simulink model "RNEDynamics"  (R2022b)
settings: Solver=ode23  StartTime=0.0  StopTime=tSim  RelTol=1e-3
values from neighbouring files (symbols this model uses):
  KdInner = 20 * eye(6)    [main.m]    (also in mainJoint.m = 40 * eye(6))
  KpInner = 4 * eye(6)    [main.m]    (also in mainJoint.m)
  qdotIC = [0, 0, 0, 0, 0, 0]'    [mainJoint.m]
  qIC = theta0'    [mainJoint.m]
  Robot = SerialLink(L)    [main.m]    (also in mainJoint.m)
undefined symbols (not defined in the file or in its folder): calcTorques, manipulatorPlant
libraries: sldrtlib x1
settings Model: Creator=Hunter  LastModifiedBy=Hunter
settings HardwareCC: ProdBitPerLong=64  ProdHWDeviceType=Intel->x86-64 (Linux 64)
settings RTWCC: Description=Simulink Desktop Real-Time  SystemTargetFile=sldrt.tlc  TemplateMakefile=sldrt.tmf  RTWCompilerOptimization=on
settings CodeAppCC: MaxIdLength=95
settings SimulinkDesktopRealTimeCC: TargetLibSuffix=_sldrt.a  TargetPreCompLibLocation=C:\Program Files\MATLAB\R2022b\toolbox\sldrt\lib\win64

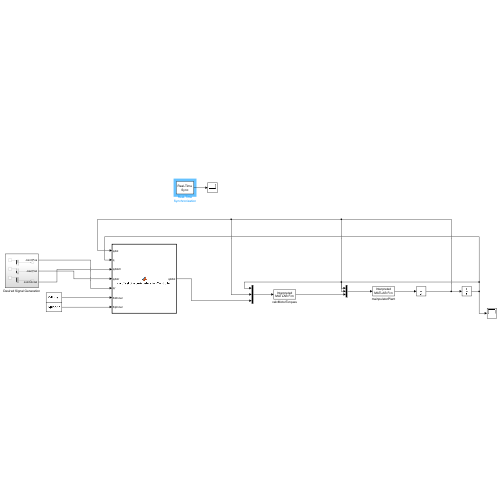
[thumbnail: Simulink's stored preview of the top-level diagram]
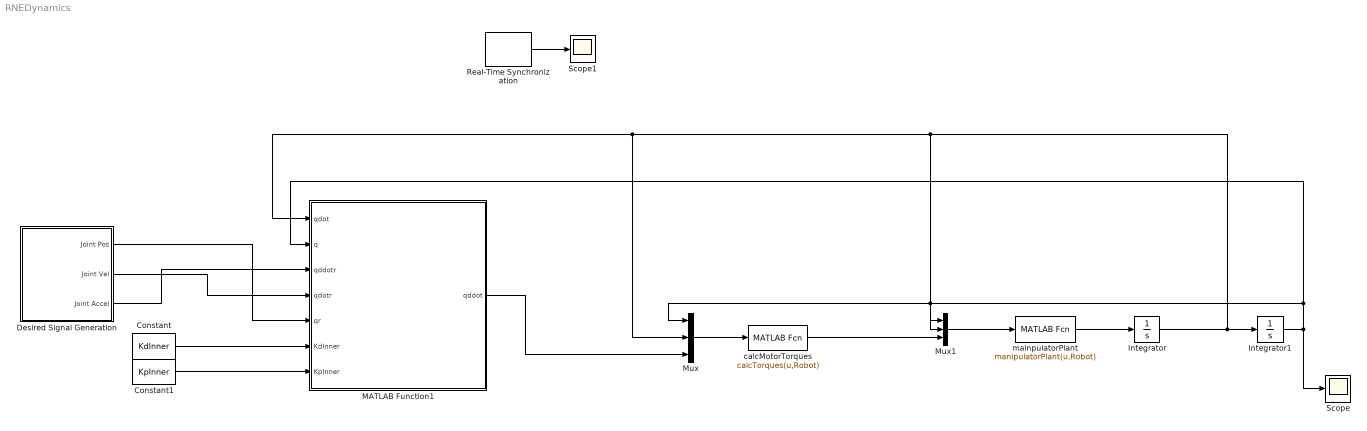
== system RNEDynamics ==
  Constant : Constant  Value=KdInner
  Constant1 : Constant  Value=KpInner
  Desired Signal Generation : Subsystem
  Integrator : Integrator  InitialCondition=qdotIC
  Integrator1 : Integrator  InitialCondition=qIC
  MATLAB Function1 : MATLAB Function  TreatAsAtomicUnit=on
  Mux : Mux  Inputs=3
  Mux1 : Mux  Inputs=3
  Real-Time Synchronization : sldrtlib/Real-Time Synchronization  SampleTime=1  MaxMissedTicks=inf  ShowMissedTicks=on  YieldWhenWaiting=off
  Scope : Scope
  Scope1 : Scope
  calcMotorTorques : MATLABFcn  MATLABFcn=calcTorques(u,Robot)  OutputDimensions=6  Output1D=off
  mainpulatorPlant : MATLABFcn  MATLABFcn=manipulatorPlant(u,Robot)
  wires:
  Desired Signal Generation/3(Joint Accel) -> MATLAB Function1/3(qddotr)
  Desired Signal Generation/2(Joint Vel) -> MATLAB Function1/4(qdotr)
  Desired Signal Generation/1(Joint Pos) -> MATLAB Function1/5(qr)
  Constant/1 -> MATLAB Function1/6(KdInner)
  Constant1/1 -> MATLAB Function1/7(KpInner)
  Mux/1 -> calcMotorTorques/1
  MATLAB Function1/1(qddot) -> Mux/3
  Mux1/1 -> mainpulatorPlant/1
  calcMotorTorques/1 -> Mux1/3
  mainpulatorPlant/1 -> Integrator/1
  Integrator/1 -> Mux1/2, Mux/2, MATLAB Function1/1(qdot), Integrator1/1
  Integrator1/1 -> Scope/1, MATLAB Function1/2(q), Mux1/1, Mux/1
  Real-Time Synchronization/1 -> Scope1/1

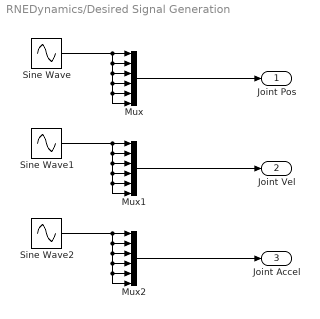
== system RNEDynamics/Desired Signal Generation ==
  Mux : Mux  Inputs=6
  Mux1 : Mux  Inputs=6
  Mux2 : Mux  Inputs=6
  Sine Wave : Sin  Amplitude=10  SampleTime=0
  Sine Wave1 : Sin  Amplitude=10  Phase=pi/2  SampleTime=0
  Sine Wave2 : Sin  Amplitude=-10  SampleTime=0
  Joint Pos : Outport
  Joint Vel : Outport  Port=2
  Joint Accel : Outport  Port=3
  wires:
  Sine Wave/1 -> Mux/6, Mux/5, Mux/4, Mux/3, Mux/2, Mux/1
  Sine Wave1/1 -> Mux1/6, Mux1/5, Mux1/4, Mux1/3, Mux1/2, Mux1/1
  Sine Wave2/1 -> Mux2/6, Mux2/5, Mux2/4, Mux2/3, Mux2/2, Mux2/1
  Mux2/1 -> Joint Accel/1
  Mux1/1 -> Joint Vel/1
  Mux/1 -> Joint Pos/1

== matlab function RNEDynamics/MATLAB Function1 ==
  data: qdot input; qddot output; q input; qddotr input; qdotr input; qr input; KdInner input; KpInner input
function qddot = calcTaskSpaceAccelerationController(qdot,q,qddotr,qdotr,qr,KdInner,KpInner)

qddot = (qddotr - KdInner * (qdot-qdotr) - KpInner * (q - qr));
